simulink model "case3"  (R2024b)
settings: Solver=FixedStepAuto  StartTime=0  StopTime=1  FixedStep=1e-7  RelTol=1e-3
values from neighbouring files (symbols this model uses):
  SG_D_1_D = 0.01056    [IEEE9_case_parameters.m]    (also in case1_parameters.m; case2_parameters.m; case3_parameters.m; case4_parameters.m)
  SG_D_1_EnableSaturation = 0    [IEEE9_case_parameters.m]    (also in case1_parameters.m; case2_parameters.m; case3_parameters.m; case4_parameters.m)
  SG_D_1_f0 = 60    [IEEE9_case_parameters.m]    (also in case1_parameters.m; case2_parameters.m; case3_parameters.m; case4_parameters.m)
  SG_D_1_H = 7.5    [IEEE9_case_parameters.m]    (also in case1_parameters.m; case2_parameters.m; case3_parameters.m; case4_parameters.m)
  SG_D_1_K_A = 20    [IEEE9_case_parameters.m]    (also in case1_parameters.m; case2_parameters.m; case3_parameters.m; case4_parameters.m)
  SG_D_1_K_E = 1.000000e+1    (= 10)    [IEEE9_case_parameters.m]    (also in case1_parameters.m; case2_parameters.m; case3_parameters.m; case4_parameters.m)
  SG_D_1_K_F = 2.363    [IEEE9_case_parameters.m]    (also in case1_parameters.m; case2_parameters.m; case3_parameters.m; case4_parameters.m)
  SG_D_1_K_s = 0.5    [IEEE9_case_parameters.m]    (also in case1_parameters.m = 5; case2_parameters.m = 5; case3_parameters.m = 5; case4_parameters.m = 5)
  SG_D_1_R_a = 0.001088    [IEEE9_case_parameters.m]    (also in case1_parameters.m; case2_parameters.m; case3_parameters.m; case4_parameters.m)
  SG_D_1_S_A = 1    [IEEE9_case_parameters.m]    (also in case1_parameters.m; case2_parameters.m; case3_parameters.m; case4_parameters.m)
  SG_D_1_S_B = 0.103    [IEEE9_case_parameters.m]    (also in case1_parameters.m; case2_parameters.m; case3_parameters.m; case4_parameters.m)
  SG_D_1_S_N = 10.659857    [IEEE9_case_parameters.m]    (also in case1_parameters.m; case2_parameters.m; case3_parameters.m; case4_parameters.m)
  SG_D_1_SpeedPara = 200    [IEEE9_case_parameters.m]    (also in case1_parameters.m; case2_parameters.m; case3_parameters.m; case4_parameters.m)
  SG_D_1_T_0 = 0.720173    [IEEE9_case_parameters.m]    (also in case1_parameters.m = 0.755522; case2_parameters.m = 0.808931; case3_parameters.m = 0.869402; case4_parameters.m = 0.729316)
  SG_D_1_T_1 = 0.3    [IEEE9_case_parameters.m]    (also in case1_parameters.m; case2_parameters.m; case3_parameters.m; case4_parameters.m)
  SG_D_1_T_2 = 0.05    [IEEE9_case_parameters.m]    (also in case1_parameters.m; case2_parameters.m; case3_parameters.m; case4_parameters.m)
  SG_D_1_T_3 = 0.02    [IEEE9_case_parameters.m]    (also in case1_parameters.m; case2_parameters.m; case3_parameters.m; case4_parameters.m)
  SG_D_1_T_4 = 0.005    [IEEE9_case_parameters.m]    (also in case1_parameters.m; case2_parameters.m; case3_parameters.m; case4_parameters.m)
  SG_D_1_T_A = 0.02    [IEEE9_case_parameters.m]    (also in case1_parameters.m; case2_parameters.m; case3_parameters.m; case4_parameters.m)
  SG_D_1_T_dd = 8.000000e+0    (= 8)    [IEEE9_case_parameters.m]    (also in case1_parameters.m; case2_parameters.m; case3_parameters.m; case4_parameters.m)
  SG_D_1_T_ddd = 0.04    [IEEE9_case_parameters.m]    (also in case1_parameters.m; case2_parameters.m; case3_parameters.m; case4_parameters.m)
  SG_D_1_T_E = 0.314    [IEEE9_case_parameters.m]    (also in case1_parameters.m; case2_parameters.m; case3_parameters.m; case4_parameters.m)
  SG_D_1_T_F = 0.35    [IEEE9_case_parameters.m]    (also in case1_parameters.m; case2_parameters.m; case3_parameters.m; case4_parameters.m)
  SG_D_1_T_qd = 0.8    [IEEE9_case_parameters.m]    (also in case1_parameters.m; case2_parameters.m; case3_parameters.m; case4_parameters.m)
  SG_D_1_T_qdd = 0.02    [IEEE9_case_parameters.m]    (also in case1_parameters.m; case2_parameters.m; case3_parameters.m; case4_parameters.m)
  SG_D_1_T_speed = 0.1    [IEEE9_case_parameters.m]    (also in case1_parameters.m = 200; case2_parameters.m = 200; case3_parameters.m = 200; case4_parameters.m = 200)
  SG_D_1_T_w = 0.5    [IEEE9_case_parameters.m]    (also in case1_parameters.m; case2_parameters.m; case3_parameters.m; case4_parameters.m)
  SG_D_1_V_ref = 1.990276    [IEEE9_case_parameters.m]    (also in case1_parameters.m = 2.042296; case2_parameters.m = 2.051388; case3_parameters.m = 2.089584; case4_parameters.m = 2.01845)
  SG_D_1_w_ref = 376.991118    [IEEE9_case_parameters.m]    (also in case1_parameters.m; case2_parameters.m; case3_parameters.m; case4_parameters.m)
  SG_D_1_wb = 6.000000e+1    (= 60)    [IEEE9_case_parameters.m]    (also in case1_parameters.m; case2_parameters.m; case3_parameters.m; case4_parameters.m)
  SG_D_1_x_d = 1.9    [IEEE9_case_parameters.m]    (also in case1_parameters.m; case2_parameters.m; case3_parameters.m; case4_parameters.m)
  SG_D_1_x_dd = 0.302    [IEEE9_case_parameters.m]    (also in case1_parameters.m; case2_parameters.m; case3_parameters.m; case4_parameters.m)
  SG_D_1_x_ddd = 0.204    [IEEE9_case_parameters.m]    (also in case1_parameters.m; case2_parameters.m; case3_parameters.m; case4_parameters.m)
  SG_D_1_x_l = 0.05    [IEEE9_case_parameters.m]    (also in case1_parameters.m; case2_parameters.m; case3_parameters.m; case4_parameters.m)
  SG_D_1_x_q = 1.3    [IEEE9_case_parameters.m]    (also in case1_parameters.m; case2_parameters.m; case3_parameters.m; case4_parameters.m)
  SG_D_1_x_qd = 0.5    [IEEE9_case_parameters.m]    (also in case1_parameters.m; case2_parameters.m; case3_parameters.m; case4_parameters.m)
  SG_D_1_x_qdd = 0.3    [IEEE9_case_parameters.m]    (also in case1_parameters.m; case2_parameters.m; case3_parameters.m; case4_parameters.m)
  SG_D_2_D = 0.02    [IEEE9_case_parameters.m]    (also in case1_parameters.m; case2_parameters.m; case3_parameters.m; case4_parameters.m)
  SG_D_2_EnableSaturation = 0    [IEEE9_case_parameters.m]    (also in case1_parameters.m; case2_parameters.m; case3_parameters.m; case4_parameters.m)
  SG_D_2_f0 = 60    [IEEE9_case_parameters.m]    (also in case1_parameters.m; case2_parameters.m; case3_parameters.m; case4_parameters.m)
  SG_D_2_H = 8.000000e+0    (= 8)    [IEEE9_case_parameters.m]    (also in case1_parameters.m; case2_parameters.m; case3_parameters.m; case4_parameters.m)
  SG_D_2_K_A = 20    [IEEE9_case_parameters.m]    (also in case1_parameters.m; case2_parameters.m; case3_parameters.m; case4_parameters.m)
  SG_D_2_K_E = 1.000000e+1    (= 10)    [IEEE9_case_parameters.m]    (also in case1_parameters.m; case2_parameters.m; case3_parameters.m; case4_parameters.m)
  SG_D_2_K_F = 2.363    [IEEE9_case_parameters.m]    (also in case1_parameters.m; case2_parameters.m; case3_parameters.m; case4_parameters.m)
  SG_D_2_K_s = 0.5    [IEEE9_case_parameters.m]    (also in case1_parameters.m = 4; case2_parameters.m = 4; case3_parameters.m = 4; case4_parameters.m = 4)
  SG_D_2_R_a = 0.001088    [IEEE9_case_parameters.m]    (also in case1_parameters.m; case2_parameters.m; case3_parameters.m; case4_parameters.m)
  SG_D_2_S_A = 1    [IEEE9_case_parameters.m]    (also in case1_parameters.m; case2_parameters.m; case3_parameters.m; case4_parameters.m)
  SG_D_2_S_B = 0.103    [IEEE9_case_parameters.m]    (also in case1_parameters.m; case2_parameters.m; case3_parameters.m; case4_parameters.m)
  SG_D_2_S_N = 10.659857    [IEEE9_case_parameters.m]    (also in case1_parameters.m; case2_parameters.m; case3_parameters.m; case4_parameters.m)
  SG_D_2_SpeedPara = 200    [IEEE9_case_parameters.m]    (also in case1_parameters.m; case2_parameters.m; case3_parameters.m; case4_parameters.m)
  SG_D_2_T_0 = 1.632913    [IEEE9_case_parameters.m]    (also in case1_parameters.m = 1.632925; case2_parameters.m = 1.632915; case3_parameters.m = 1.632914; case4_parameters.m = 1.632927)
  SG_D_2_T_1 = 0.2    [IEEE9_case_parameters.m]    (also in case1_parameters.m; case2_parameters.m; case3_parameters.m; case4_parameters.m)
  SG_D_2_T_2 = 0.05    [IEEE9_case_parameters.m]    (also in case1_parameters.m; case2_parameters.m; case3_parameters.m; case4_parameters.m)
  SG_D_2_T_3 = 0.02    [IEEE9_case_parameters.m]    (also in case1_parameters.m; case2_parameters.m; case3_parameters.m; case4_parameters.m)
  SG_D_2_T_4 = 0.005    [IEEE9_case_parameters.m]    (also in case1_parameters.m; case2_parameters.m; case3_parameters.m; case4_parameters.m)
  SG_D_2_T_A = 0.02    [IEEE9_case_parameters.m]    (also in case1_parameters.m; case2_parameters.m; case3_parameters.m; case4_parameters.m)
  SG_D_2_T_dd = 7.9    [IEEE9_case_parameters.m]    (also in case1_parameters.m; case2_parameters.m; case3_parameters.m; case4_parameters.m)
  SG_D_2_T_ddd = 0.04    [IEEE9_case_parameters.m]    (also in case1_parameters.m; case2_parameters.m; case3_parameters.m; case4_parameters.m)
  SG_D_2_T_E = 0.314    [IEEE9_case_parameters.m]    (also in case1_parameters.m; case2_parameters.m; case3_parameters.m; case4_parameters.m)
  SG_D_2_T_F = 0.35    [IEEE9_case_parameters.m]    (also in case1_parameters.m; case2_parameters.m; case3_parameters.m; case4_parameters.m)
  SG_D_2_T_qd = 0.8    [IEEE9_case_parameters.m]    (also in case1_parameters.m; case2_parameters.m; case3_parameters.m; case4_parameters.m)
  SG_D_2_T_qdd = 0.015    [IEEE9_case_parameters.m]    (also in case1_parameters.m; case2_parameters.m; case3_parameters.m; case4_parameters.m)
  SG_D_2_T_speed = 0.1    [IEEE9_case_parameters.m]    (also in case1_parameters.m = 150; case2_parameters.m = 150; case3_parameters.m = 150; case4_parameters.m = 150)
  SG_D_2_T_w = 0.35    [IEEE9_case_parameters.m]    (also in case1_parameters.m; case2_parameters.m; case3_parameters.m; case4_parameters.m)
  SG_D_2_V_ref = 2.58547    [IEEE9_case_parameters.m]    (also in case1_parameters.m = 2.597896; case2_parameters.m = 2.587136; case3_parameters.m = 2.586042; case4_parameters.m = 2.599679)
  SG_D_2_w_ref = 376.991118    [IEEE9_case_parameters.m]    (also in case1_parameters.m; case2_parameters.m; case3_parameters.m; case4_parameters.m)
  SG_D_2_wb = 6.000000e+1    (= 60)    [IEEE9_case_parameters.m]    (also in case1_parameters.m; case2_parameters.m; case3_parameters.m; case4_parameters.m)
  SG_D_2_x_d = 1.8    [IEEE9_case_parameters.m]    (also in case1_parameters.m; case2_parameters.m; case3_parameters.m; case4_parameters.m)
  SG_D_2_x_dd = 0.302    [IEEE9_case_parameters.m]    (also in case1_parameters.m; case2_parameters.m; case3_parameters.m; case4_parameters.m)
  SG_D_2_x_ddd = 0.204    [IEEE9_case_parameters.m]    (also in case1_parameters.m; case2_parameters.m; case3_parameters.m; case4_parameters.m)
  SG_D_2_x_l = 0.05    [IEEE9_case_parameters.m]    (also in case1_parameters.m; case2_parameters.m; case3_parameters.m; case4_parameters.m)
  SG_D_2_x_q = 1.25    [IEEE9_case_parameters.m]    (also in case1_parameters.m; case2_parameters.m; case3_parameters.m; case4_parameters.m)
  SG_D_2_x_qd = 0.5    [IEEE9_case_parameters.m]    (also in case1_parameters.m; case2_parameters.m; case3_parameters.m; case4_parameters.m)
  SG_D_2_x_qdd = 0.3    [IEEE9_case_parameters.m]    (also in case1_parameters.m; case2_parameters.m; case3_parameters.m; case4_parameters.m)
  SG_D_3_D = 0.02    [IEEE9_case_parameters.m]    (also in case1_parameters.m; case2_parameters.m; case3_parameters.m; case4_parameters.m)
  SG_D_3_EnableSaturation = 0    [IEEE9_case_parameters.m]    (also in case1_parameters.m; case2_parameters.m; case3_parameters.m; case4_parameters.m)
  SG_D_3_f0 = 60    [IEEE9_case_parameters.m]    (also in case1_parameters.m; case2_parameters.m; case3_parameters.m; case4_parameters.m)
  SG_D_3_H = 7.7    [IEEE9_case_parameters.m]    (also in case1_parameters.m; case2_parameters.m; case3_parameters.m; case4_parameters.m)
  SG_D_3_K_A = 20    [IEEE9_case_parameters.m]    (also in case1_parameters.m; case2_parameters.m; case3_parameters.m; case4_parameters.m)
  SG_D_3_K_E = 1.000000e+1    (= 10)    [IEEE9_case_parameters.m]    (also in case1_parameters.m; case2_parameters.m; case3_parameters.m; case4_parameters.m)
  SG_D_3_K_F = 2.363    [IEEE9_case_parameters.m]    (also in case1_parameters.m; case2_parameters.m; case3_parameters.m; case4_parameters.m)
  SG_D_3_K_s = 0.2    [IEEE9_case_parameters.m]    (also in case1_parameters.m = 2; case2_parameters.m = 2; case3_parameters.m = 2; case4_parameters.m = 2)
  SG_D_3_R_a = 0.001088    [IEEE9_case_parameters.m]    (also in case1_parameters.m; case2_parameters.m; case3_parameters.m; case4_parameters.m)
  SG_D_3_S_A = 1    [IEEE9_case_parameters.m]    (also in case1_parameters.m; case2_parameters.m; case3_parameters.m; case4_parameters.m)
  SG_D_3_S_B = 0.103    [IEEE9_case_parameters.m]    (also in case1_parameters.m; case2_parameters.m; case3_parameters.m; case4_parameters.m)
  SG_D_3_S_N = 10.659857    [IEEE9_case_parameters.m]    (also in case1_parameters.m; case2_parameters.m; case3_parameters.m; case4_parameters.m)
  SG_D_3_SpeedPara = 200    [IEEE9_case_parameters.m]    (also in case1_parameters.m; case2_parameters.m; case3_parameters.m; case4_parameters.m)
  SG_D_3_T_0 = 0.850788    [IEEE9_case_parameters.m]    (also in case1_parameters.m = 0.850786; case2_parameters.m = 0.850787; case3_parameters.m; case4_parameters.m = 0.850786)
  SG_D_3_T_1 = 0.2    [IEEE9_case_parameters.m]    (also in case1_parameters.m; case2_parameters.m; case3_parameters.m; case4_parameters.m)
  SG_D_3_T_2 = 0.05    [IEEE9_case_parameters.m]    (also in case1_parameters.m; case2_parameters.m; case3_parameters.m; case4_parameters.m)
  SG_D_3_T_3 = 0.02    [IEEE9_case_parameters.m]    (also in case1_parameters.m; case2_parameters.m; case3_parameters.m; case4_parameters.m)
  SG_D_3_T_4 = 0.005    [IEEE9_case_parameters.m]    (also in case1_parameters.m; case2_parameters.m; case3_parameters.m; case4_parameters.m)
  SG_D_3_T_A = 0.02    [IEEE9_case_parameters.m]    (also in case1_parameters.m; case2_parameters.m; case3_parameters.m; case4_parameters.m)
  SG_D_3_T_dd = 8.1    [IEEE9_case_parameters.m]    (also in case1_parameters.m; case2_parameters.m; case3_parameters.m; case4_parameters.m)
  SG_D_3_T_ddd = 0.04    [IEEE9_case_parameters.m]    (also in case1_parameters.m; case2_parameters.m; case3_parameters.m; case4_parameters.m)
  SG_D_3_T_E = 0.314    [IEEE9_case_parameters.m]    (also in case1_parameters.m; case2_parameters.m; case3_parameters.m; case4_parameters.m)
  SG_D_3_T_F = 0.35    [IEEE9_case_parameters.m]    (also in case1_parameters.m; case2_parameters.m; case3_parameters.m; case4_parameters.m)
  SG_D_3_T_qd = 0.8    [IEEE9_case_parameters.m]    (also in case1_parameters.m; case2_parameters.m; case3_parameters.m; case4_parameters.m)
  SG_D_3_T_qdd = 0.015    [IEEE9_case_parameters.m]    (also in case1_parameters.m; case2_parameters.m; case3_parameters.m; case4_parameters.m)
  SG_D_3_T_speed = 0.1    [IEEE9_case_parameters.m]    (also in case1_parameters.m = 180; case2_parameters.m = 180; case3_parameters.m = 180; case4_parameters.m = 180)
  SG_D_3_T_w = 0.4    [IEEE9_case_parameters.m]    (also in case1_parameters.m; case2_parameters.m; case3_parameters.m; case4_parameters.m)
  SG_D_3_V_ref = 1.892727    [IEEE9_case_parameters.m]    (also in case1_parameters.m = 1.906439; case2_parameters.m = 1.895535; case3_parameters.m = 1.892105; case4_parameters.m = 1.906598)
  SG_D_3_w_ref = 376.991118    [IEEE9_case_parameters.m]    (also in case1_parameters.m; case2_parameters.m; case3_parameters.m; case4_parameters.m)
  SG_D_3_wb = 6.000000e+1    (= 60)    [IEEE9_case_parameters.m]    (also in case1_parameters.m; case2_parameters.m; case3_parameters.m; case4_parameters.m)
  SG_D_3_x_d = 1.85    [IEEE9_case_parameters.m]    (also in case1_parameters.m; case2_parameters.m; case3_parameters.m; case4_parameters.m)
  SG_D_3_x_dd = 0.302    [IEEE9_case_parameters.m]    (also in case1_parameters.m; case2_parameters.m; case3_parameters.m; case4_parameters.m)
  SG_D_3_x_ddd = 0.204    [IEEE9_case_parameters.m]    (also in case1_parameters.m; case2_parameters.m; case3_parameters.m; case4_parameters.m)
  SG_D_3_x_l = 0.05    [IEEE9_case_parameters.m]    (also in case1_parameters.m; case2_parameters.m; case3_parameters.m; case4_parameters.m)
  SG_D_3_x_q = 1.2    [IEEE9_case_parameters.m]    (also in case1_parameters.m; case2_parameters.m; case3_parameters.m; case4_parameters.m)
  SG_D_3_x_qd = 0.5    [IEEE9_case_parameters.m]    (also in case1_parameters.m; case2_parameters.m; case3_parameters.m; case4_parameters.m)
  SG_D_3_x_qdd = 0.3    [IEEE9_case_parameters.m]    (also in case1_parameters.m; case2_parameters.m; case3_parameters.m; case4_parameters.m)
(part 4 of 12)

== system case3/AC_1/d_vq_bus_7_block ==
  note: d_vq_bus_7 in case3
      | $2106.09563369148\,\mathrm{iq}_{\mathrm{bus},7}-376.991118430775\,\mathrm{vd}_{\mathrm{bus},7}$
      | Automatically generated on 2025-10-31 19:02:04 .
  Alge_iq_bus_7_9bcfd : Inport
  State_vd_bus_7_2341e : Inport  Port=2
  Constant_2106.09563369148_1523e : Constant  Value=2106.09563369148
  Constant_376.991118430775_cd95a : Constant  Value=376.991118430775
  Product_43391 : Product
  Product_ed048 : Product
  Subtract_00e21 : Sum  Inputs=+-
  Blockout_d_vq_bus_7_00412 : Outport
  wires:
  Constant_2106.09563369148_1523e/1 -> Product_ed048/1
  Product_43391/1 -> Subtract_00e21/2
  Alge_iq_bus_7_9bcfd/1 -> Product_ed048/2
  Constant_376.991118430775_cd95a/1 -> Product_43391/1
  Subtract_00e21/1 -> Blockout_d_vq_bus_7_00412/1
  State_vd_bus_7_2341e/1 -> Product_43391/2
  Product_ed048/1 -> Subtract_00e21/1

== system case3/AC_1/d_vq_bus_8_block ==
  note: d_vq_bus_8 in case3
      | $1657.10381727813\,\mathrm{iq}_{\mathrm{bus},8}-376.991118430775\,\mathrm{vd}_{\mathrm{bus},8}$
      | Automatically generated on 2025-10-31 19:02:06 .
  Alge_iq_bus_8_0043b : Inport
  State_vd_bus_8_4778f : Inport  Port=2
  Constant_1657.10381727813_76750 : Constant  Value=1657.10381727813
  Constant_376.991118430775_a4e06 : Constant  Value=376.991118430775
  Product_09aa2 : Product
  Product_80b30 : Product
  Subtract_72ad1 : Sum  Inputs=+-
  Blockout_d_vq_bus_8_7125c : Outport
  wires:
  Constant_1657.10381727813_76750/1 -> Product_09aa2/1
  Constant_376.991118430775_a4e06/1 -> Product_80b30/1
  Alge_iq_bus_8_0043b/1 -> Product_09aa2/2
  State_vd_bus_8_4778f/1 -> Product_80b30/2
  Product_09aa2/1 -> Subtract_72ad1/1
  Product_80b30/1 -> Subtract_72ad1/2
  Subtract_72ad1/1 -> Blockout_d_vq_bus_8_7125c/1

== system case3/AC_1/d_vq_bus_9_block ==
  note: d_vq_bus_9 in case3
      | $1564.27849971276\,\mathrm{iq}_{\mathrm{bus},9}-376.991118430775\,\mathrm{vd}_{\mathrm{bus},9}$
      | Automatically generated on 2025-10-31 19:02:07 .
  Alge_iq_bus_9_e4ae9 : Inport
  State_vd_bus_9_0824c : Inport  Port=2
  Constant_1564.27849971276_a5fe3 : Constant  Value=1564.27849971276
  Constant_376.991118430775_65cab : Constant  Value=376.991118430775
  Product_26de2 : Product
  Product_50707 : Product
  Subtract_bc7f1 : Sum  Inputs=+-
  Blockout_d_vq_bus_9_e5b12 : Outport
  wires:
  Constant_1564.27849971276_a5fe3/1 -> Product_50707/1
  Constant_376.991118430775_65cab/1 -> Product_26de2/1
  Alge_iq_bus_9_e4ae9/1 -> Product_50707/2
  State_vd_bus_9_0824c/1 -> Product_26de2/2
  Product_50707/1 -> Subtract_bc7f1/1
  Product_26de2/1 -> Subtract_bc7f1/2
  Subtract_bc7f1/1 -> Blockout_d_vq_bus_9_e5b12/1

== system case3/AC_1/id_bus_1_block ==
  note: id_bus_1 in case3
      | $\mathrm{id}_{\mathrm{SG},D,1}-\mathrm{id}_{\mathrm{line},1,4}$
      | Automatically generated on 2025-10-31 19:02:38 .
  Input_id_SG_D_1_696b1 : Inport
  State_id_line_1_4_e72f3 : Inport  Port=2
  Subtract_53e99 : Sum  Inputs=+-
  Blockout_id_bus_1_4a65c : Outport
  wires:
  Input_id_SG_D_1_696b1/1 -> Subtract_53e99/1
  State_id_line_1_4_e72f3/1 -> Subtract_53e99/2
  Subtract_53e99/1 -> Blockout_id_bus_1_4a65c/1

== system case3/AC_1/id_bus_2_block ==
  note: id_bus_2 in case3
      | $\mathrm{id}_{\mathrm{SG},D,2}+\mathrm{id}_{\mathrm{line},8,2}$
      | Automatically generated on 2025-10-31 19:02:40 .
  Input_id_SG_D_2_bafef : Inport
  State_id_line_8_2_6b5a6 : Inport  Port=2
  Add_c2829 : Sum
  Blockout_id_bus_2_bddd5 : Outport
  wires:
  Input_id_SG_D_2_bafef/1 -> Add_c2829/1
  State_id_line_8_2_6b5a6/1 -> Add_c2829/2
  Add_c2829/1 -> Blockout_id_bus_2_bddd5/1

== system case3/AC_1/id_bus_3_block ==
  note: id_bus_3 in case3
      | $\mathrm{id}_{\mathrm{SG},D,3}-\mathrm{id}_{\mathrm{line},3,6}$
      | Automatically generated on 2025-10-31 19:02:43 .
  Input_id_SG_D_3_6c44f : Inport
  State_id_line_3_6_571a6 : Inport  Port=2
  Subtract_f2fe0 : Sum  Inputs=+-
  Blockout_id_bus_3_5b536 : Outport
  wires:
  Input_id_SG_D_3_6c44f/1 -> Subtract_f2fe0/1
  State_id_line_3_6_571a6/1 -> Subtract_f2fe0/2
  Subtract_f2fe0/1 -> Blockout_id_bus_3_5b536/1

== system case3/AC_1/id_bus_4_block ==
  note: id_bus_4 in case3
      | $\mathrm{id}_{\mathrm{line},1,4}-\mathrm{id}_{\mathrm{line},4,5}+\mathrm{id}_{\mathrm{line},9,4}$
      | Automatically generated on 2025-10-31 19:02:44 .
  State_id_line_1_4_bd9f3 : Inport
  State_id_line_4_5_71002 : Inport  Port=2
  State_id_line_9_4_dd8eb : Inport  Port=3
  Add_de6d1 : Sum
  Subtract_ec270 : Sum  Inputs=+-
  Blockout_id_bus_4_47d2f : Outport
  wires:
  State_id_line_9_4_dd8eb/1 -> Add_de6d1/2
  State_id_line_1_4_bd9f3/1 -> Subtract_ec270/1
  State_id_line_4_5_71002/1 -> Subtract_ec270/2
  Subtract_ec270/1 -> Add_de6d1/1
  Add_de6d1/1 -> Blockout_id_bus_4_47d2f/1

== system case3/AC_1/id_bus_5_block ==
  note: id_bus_5 in case3
      | $\mathrm{id}_{\mathrm{line},4,5}-\mathrm{id}_{\mathrm{load},5}-\mathrm{id}_{\mathrm{line},5,6}$
      | Automatically generated on 2025-10-31 19:02:46 .
  State_id_load_5_b6667 : Inport
  State_id_line_4_5_78e66 : Inport  Port=2
  State_id_line_5_6_8fb3f : Inport  Port=3
  Add_36a5e : Sum
  Constant_-1_8506f : Constant  Value=-1
  Product_690f2 : Product
  Subtract_ac2bb : Sum  Inputs=+-
  Blockout_id_bus_5_0f46c : Outport
  wires:
  Subtract_ac2bb/1 -> Blockout_id_bus_5_0f46c/1
  State_id_line_4_5_78e66/1 -> Add_36a5e/2
  Constant_-1_8506f/1 -> Product_690f2/1
  Add_36a5e/1 -> Subtract_ac2bb/1
  State_id_load_5_b6667/1 -> Product_690f2/2
  Product_690f2/1 -> Add_36a5e/1
  State_id_line_5_6_8fb3f/1 -> Subtract_ac2bb/2

== system case3/AC_1/id_bus_6_block ==
  note: id_bus_6 in case3
      | $\mathrm{id}_{\mathrm{line},3,6}+\mathrm{id}_{\mathrm{line},5,6}-\mathrm{id}_{\mathrm{line},6,7}$
      | Automatically generated on 2025-10-31 19:02:47 .
  State_id_line_3_6_c6af3 : Inport
  State_id_line_5_6_cc1e8 : Inport  Port=2
  State_id_line_6_7_32134 : Inport  Port=3
  Add_59c7e : Sum
  Subtract_31bf1 : Sum  Inputs=+-
  Blockout_id_bus_6_05d15 : Outport
  wires:
  State_id_line_6_7_32134/1 -> Subtract_31bf1/2
  State_id_line_3_6_c6af3/1 -> Add_59c7e/1
  State_id_line_5_6_cc1e8/1 -> Add_59c7e/2
  Add_59c7e/1 -> Subtract_31bf1/1
  Subtract_31bf1/1 -> Blockout_id_bus_6_05d15/1

== system case3/AC_1/id_bus_7_block ==
  note: id_bus_7 in case3
      | $\mathrm{id}_{\mathrm{line},6,7}-\mathrm{id}_{\mathrm{load},7}-\mathrm{id}_{\mathrm{line},7,8}$
      | Automatically generated on 2025-10-31 19:02:49 .
  State_id_load_7_37f76 : Inport
  State_id_line_6_7_64680 : Inport  Port=2
  State_id_line_7_8_85cde : Inport  Port=3
  Add_ba5f6 : Sum
  Constant_-1_f6e4f : Constant  Value=-1
  Product_2a424 : Product
  Subtract_4cf74 : Sum  Inputs=+-
  Blockout_id_bus_7_20b6b : Outport
  wires:
  Subtract_4cf74/1 -> Blockout_id_bus_7_20b6b/1
  State_id_line_6_7_64680/1 -> Add_ba5f6/2
  Constant_-1_f6e4f/1 -> Product_2a424/1
  Add_ba5f6/1 -> Subtract_4cf74/1
  State_id_load_7_37f76/1 -> Product_2a424/2
  Product_2a424/1 -> Add_ba5f6/1
  State_id_line_7_8_85cde/1 -> Subtract_4cf74/2

== system case3/AC_1/id_bus_8_block ==
  note: id_bus_8 in case3
      | $\mathrm{id}_{\mathrm{line},7,8}-\mathrm{id}_{\mathrm{line},8,2}-\mathrm{id}_{\mathrm{line},8,9}$
      | Automatically generated on 2025-10-31 19:02:51 .
  State_id_line_7_8_e2cc9 : Inport
  State_id_line_8_2_3e7ba : Inport  Port=2
  State_id_line_8_9_302ee : Inport  Port=3
  Subtract_27381 : Sum  Inputs=+-
  Subtract_b9667 : Sum  Inputs=+-
  Blockout_id_bus_8_01350 : Outport
  wires:
  State_id_line_8_9_302ee/1 -> Subtract_b9667/2
  State_id_line_7_8_e2cc9/1 -> Subtract_27381/1
  State_id_line_8_2_3e7ba/1 -> Subtract_27381/2
  Subtract_27381/1 -> Subtract_b9667/1
  Subtract_b9667/1 -> Blockout_id_bus_8_01350/1

== system case3/AC_1/id_bus_9_block ==
  note: id_bus_9 in case3
      | $\mathrm{id}_{\mathrm{line},8,9}-\mathrm{id}_{\mathrm{load},9}-\mathrm{id}_{\mathrm{line},9,4}$
      | Automatically generated on 2025-10-31 19:02:52 .
  State_id_load_9_08adc : Inport
  State_id_line_8_9_ceed5 : Inport  Port=2
  State_id_line_9_4_1728f : Inport  Port=3
  Add_64fa5 : Sum
  Constant_-1_2f2f1 : Constant  Value=-1
  Product_af254 : Product
  Subtract_1fc9b : Sum  Inputs=+-
  Blockout_id_bus_9_70dbc : Outport
  wires:
  Subtract_1fc9b/1 -> Blockout_id_bus_9_70dbc/1
  State_id_line_8_9_ceed5/1 -> Add_64fa5/2
  Constant_-1_2f2f1/1 -> Product_af254/1
  Add_64fa5/1 -> Subtract_1fc9b/1
  State_id_load_9_08adc/1 -> Product_af254/2
  Product_af254/1 -> Add_64fa5/1
  State_id_line_9_4_1728f/1 -> Subtract_1fc9b/2

== system case3/AC_1/iq_bus_1_block ==
  note: iq_bus_1 in case3
      | $\mathrm{iq}_{\mathrm{SG},D,1}-\mathrm{iq}_{\mathrm{line},1,4}$
      | Automatically generated on 2025-10-31 19:02:38 .
  Input_iq_SG_D_1_691df : Inport
  State_iq_line_1_4_8b10a : Inport  Port=2
  Subtract_bf583 : Sum  Inputs=+-
  Blockout_iq_bus_1_cefb8 : Outport
  wires:
  Input_iq_SG_D_1_691df/1 -> Subtract_bf583/1
  State_iq_line_1_4_8b10a/1 -> Subtract_bf583/2
  Subtract_bf583/1 -> Blockout_iq_bus_1_cefb8/1

== system case3/AC_1/iq_bus_2_block ==
  note: iq_bus_2 in case3
      | $\mathrm{iq}_{\mathrm{SG},D,2}+\mathrm{iq}_{\mathrm{line},8,2}$
      | Automatically generated on 2025-10-31 19:02:41 .
  Input_iq_SG_D_2_ed99c : Inport
  State_iq_line_8_2_3621d : Inport  Port=2
  Add_92b39 : Sum
  Blockout_iq_bus_2_c2560 : Outport
  wires:
  Input_iq_SG_D_2_ed99c/1 -> Add_92b39/1
  State_iq_line_8_2_3621d/1 -> Add_92b39/2
  Add_92b39/1 -> Blockout_iq_bus_2_c2560/1

== system case3/AC_1/iq_bus_3_block ==
  note: iq_bus_3 in case3
      | $\mathrm{iq}_{\mathrm{SG},D,3}-\mathrm{iq}_{\mathrm{line},3,6}$
      | Automatically generated on 2025-10-31 19:02:43 .
  Input_iq_SG_D_3_dee65 : Inport
  State_iq_line_3_6_61dd2 : Inport  Port=2
  Subtract_e728d : Sum  Inputs=+-
  Blockout_iq_bus_3_7f48b : Outport
  wires:
  Input_iq_SG_D_3_dee65/1 -> Subtract_e728d/1
  State_iq_line_3_6_61dd2/1 -> Subtract_e728d/2
  Subtract_e728d/1 -> Blockout_iq_bus_3_7f48b/1

== system case3/AC_1/iq_bus_4_block ==
  note: iq_bus_4 in case3
      | $\mathrm{iq}_{\mathrm{line},1,4}-\mathrm{iq}_{\mathrm{line},4,5}+\mathrm{iq}_{\mathrm{line},9,4}$
      | Automatically generated on 2025-10-31 19:02:45 .
  State_iq_line_1_4_b88bb : Inport
  State_iq_line_4_5_adb37 : Inport  Port=2
  State_iq_line_9_4_3e12c : Inport  Port=3
  Add_1fb56 : Sum
  Subtract_2b2df : Sum  Inputs=+-
  Blockout_iq_bus_4_14ae7 : Outport
  wires:
  State_iq_line_1_4_b88bb/1 -> Subtract_2b2df/1
  State_iq_line_4_5_adb37/1 -> Subtract_2b2df/2
  Subtract_2b2df/1 -> Add_1fb56/1
  State_iq_line_9_4_3e12c/1 -> Add_1fb56/2
  Add_1fb56/1 -> Blockout_iq_bus_4_14ae7/1

== system case3/AC_1/iq_bus_5_block ==
  note: iq_bus_5 in case3
      | $\mathrm{iq}_{\mathrm{line},4,5}-\mathrm{iq}_{\mathrm{load},5}-\mathrm{iq}_{\mathrm{line},5,6}$
      | Automatically generated on 2025-10-31 19:02:47 .
  State_iq_load_5_2754d : Inport
  State_iq_line_4_5_89bcd : Inport  Port=2
  State_iq_line_5_6_c4019 : Inport  Port=3
  Add_c4d41 : Sum
  Constant_-1_2f333 : Constant  Value=-1
  Product_39ca3 : Product
  Subtract_68927 : Sum  Inputs=+-
  Blockout_iq_bus_5_d6d28 : Outport
  wires:
  Subtract_68927/1 -> Blockout_iq_bus_5_d6d28/1
  State_iq_line_4_5_89bcd/1 -> Add_c4d41/2
  Constant_-1_2f333/1 -> Product_39ca3/1
  State_iq_load_5_2754d/1 -> Product_39ca3/2
  Product_39ca3/1 -> Add_c4d41/1
  Add_c4d41/1 -> Subtract_68927/1
  State_iq_line_5_6_c4019/1 -> Subtract_68927/2

== system case3/AC_1/iq_bus_6_block ==
  note: iq_bus_6 in case3
      | $\mathrm{iq}_{\mathrm{line},3,6}+\mathrm{iq}_{\mathrm{line},5,6}-\mathrm{iq}_{\mathrm{line},6,7}$
      | Automatically generated on 2025-10-31 19:02:48 .
  State_iq_line_3_6_33d27 : Inport
  State_iq_line_5_6_019c6 : Inport  Port=2
  State_iq_line_6_7_054b0 : Inport  Port=3
  Add_d3aef : Sum
  Subtract_4e3ec : Sum  Inputs=+-
  Blockout_iq_bus_6_95ebc : Outport
  wires:
  State_iq_line_3_6_33d27/1 -> Add_d3aef/1
  State_iq_line_5_6_019c6/1 -> Add_d3aef/2
  Add_d3aef/1 -> Subtract_4e3ec/1
  State_iq_line_6_7_054b0/1 -> Subtract_4e3ec/2
  Subtract_4e3ec/1 -> Blockout_iq_bus_6_95ebc/1

== system case3/AC_1/iq_bus_7_block ==
  note: iq_bus_7 in case3
      | $\mathrm{iq}_{\mathrm{line},6,7}-\mathrm{iq}_{\mathrm{load},7}-\mathrm{iq}_{\mathrm{line},7,8}$
      | Automatically generated on 2025-10-31 19:02:50 .
  State_iq_load_7_960e8 : Inport
  State_iq_line_6_7_03f81 : Inport  Port=2
  State_iq_line_7_8_95be5 : Inport  Port=3
  Add_47c7b : Sum
  Constant_-1_469e3 : Constant  Value=-1
  Product_518e4 : Product
  Subtract_c0759 : Sum  Inputs=+-
  Blockout_iq_bus_7_bb486 : Outport
  wires:
  Subtract_c0759/1 -> Blockout_iq_bus_7_bb486/1
  State_iq_line_6_7_03f81/1 -> Add_47c7b/2
  Constant_-1_469e3/1 -> Product_518e4/1
  State_iq_load_7_960e8/1 -> Product_518e4/2
  Product_518e4/1 -> Add_47c7b/1
  Add_47c7b/1 -> Subtract_c0759/1
  State_iq_line_7_8_95be5/1 -> Subtract_c0759/2

== system case3/AC_1/iq_bus_8_block ==
  note: iq_bus_8 in case3
      | $\mathrm{iq}_{\mathrm{line},7,8}-\mathrm{iq}_{\mathrm{line},8,2}-\mathrm{iq}_{\mathrm{line},8,9}$
      | Automatically generated on 2025-10-31 19:02:51 .
  State_iq_line_7_8_0aaeb : Inport
  State_iq_line_8_2_60ac3 : Inport  Port=2
  State_iq_line_8_9_6619f : Inport  Port=3
  Subtract_54fe6 : Sum  Inputs=+-
  Subtract_93871 : Sum  Inputs=+-
  Blockout_iq_bus_8_33408 : Outport
  wires:
  State_iq_line_7_8_0aaeb/1 -> Subtract_54fe6/1
  State_iq_line_8_2_60ac3/1 -> Subtract_54fe6/2
  Subtract_54fe6/1 -> Subtract_93871/1
  State_iq_line_8_9_6619f/1 -> Subtract_93871/2
  Subtract_93871/1 -> Blockout_iq_bus_8_33408/1

== system case3/AC_1/iq_bus_9_block ==
  note: iq_bus_9 in case3
      | $\mathrm{iq}_{\mathrm{line},8,9}-\mathrm{iq}_{\mathrm{load},9}-\mathrm{iq}_{\mathrm{line},9,4}$
      | Automatically generated on 2025-10-31 19:02:53 .
  State_iq_load_9_56201 : Inport
  State_iq_line_8_9_f042c : Inport  Port=2
  State_iq_line_9_4_00fae : Inport  Port=3
  Add_29842 : Sum
  Constant_-1_51dab : Constant  Value=-1
  Product_ccf99 : Product
  Subtract_5ae72 : Sum  Inputs=+-
  Blockout_iq_bus_9_4e4a2 : Outport
  wires:
  Subtract_5ae72/1 -> Blockout_iq_bus_9_4e4a2/1
  State_iq_line_8_9_f042c/1 -> Add_29842/2
  Constant_-1_51dab/1 -> Product_ccf99/1
  State_iq_load_9_56201/1 -> Product_ccf99/2
  Product_ccf99/1 -> Add_29842/1
  Add_29842/1 -> Subtract_5ae72/1
  State_iq_line_9_4_00fae/1 -> Subtract_5ae72/2

== system case3/AC_1/vd_bus_1_out_block ==
  note: vd_bus_1_out in case3
      | $\mathrm{vd}_{\mathrm{bus},1}$
      | Automatically generated on 2025-10-31 19:02:37 .
  State_vd_bus_1_379f4 : Inport
  Blockout_vd_bus_1_out_2faa7 : Outport
  wires:
  State_vd_bus_1_379f4/1 -> Blockout_vd_bus_1_out_2faa7/1

== system case3/AC_1/vd_bus_2_out_block ==
  note: vd_bus_2_out in case3
      | $\mathrm{vd}_{\mathrm{bus},2}$
      | Automatically generated on 2025-10-31 19:02:39 .
  State_vd_bus_2_2714d : Inport
  Blockout_vd_bus_2_out_79f6a : Outport
  wires:
  State_vd_bus_2_2714d/1 -> Blockout_vd_bus_2_out_79f6a/1

== system case3/AC_1/vd_bus_3_out_block ==
  note: vd_bus_3_out in case3
      | $\mathrm{vd}_{\mathrm{bus},3}$
      | Automatically generated on 2025-10-31 19:02:41 .
  State_vd_bus_3_9218c : Inport
  Blockout_vd_bus_3_out_036f2 : Outport
  wires:
  State_vd_bus_3_9218c/1 -> Blockout_vd_bus_3_out_036f2/1

== system case3/AC_1/vq_bus_1_out_block ==
  note: vq_bus_1_out in case3
      | $\mathrm{vq}_{\mathrm{bus},1}$
      | Automatically generated on 2025-10-31 19:02:37 .
  State_vq_bus_1_ac5cf : Inport
  Blockout_vq_bus_1_out_b4fc0 : Outport
  wires:
  State_vq_bus_1_ac5cf/1 -> Blockout_vq_bus_1_out_b4fc0/1

== system case3/AC_1/vq_bus_2_out_block ==
  note: vq_bus_2_out in case3
      | $\mathrm{vq}_{\mathrm{bus},2}$
      | Automatically generated on 2025-10-31 19:02:39 .
  State_vq_bus_2_9d425 : Inport
  Blockout_vq_bus_2_out_740a9 : Outport
  wires:
  State_vq_bus_2_9d425/1 -> Blockout_vq_bus_2_out_740a9/1

== system case3/AC_1/vq_bus_3_out_block ==
  note: vq_bus_3_out in case3
      | $\mathrm{vq}_{\mathrm{bus},3}$
      | Automatically generated on 2025-10-31 19:02:42 .
  State_vq_bus_3_4ba96 : Inport
  Blockout_vq_bus_3_out_fa0c1 : Outport
  wires:
  State_vq_bus_3_4ba96/1 -> Blockout_vq_bus_3_out_fa0c1/1

== system case3/SG_D_1/T_e_SG_D_1_block ==
  note: T_e_SG_D_1 in case3
      | $-\frac{\psi _{d,\mathrm{SG},D,1}\,\left(\psi _{q,\mathrm{SG},D,1}+\frac{\psi _{\mathrm{gq},\mathrm{SG},D,1}\,\left(x_{l}-x_{\mathrm{qdd}}\right)}{x_{l}-x_{\mathrm{qd}}}+\frac{\psi _{\mathrm{kq},\mathrm{SG},D,1}\,\left(x_{\mathrm{qd}}-x_{\mathrm{qdd}}\right)}{x_{l}-x_{\mathrm{qd}}}\right)}{x_{\mathrm{qdd}}}-\frac{\psi _{q,\mathrm{SG},D,1}\,\left(\frac{\psi _{\mathrm{1d},\mathrm{SG},D,1}\,\left(x_{\mathrm{dd}}-x_{\mathrm{ddd}}\right)}{x_{\mathrm{dd}}-x_{l}}-\psi _{d,\mathrm{SG},D,1}+\frac{\psi _{\mathrm{fd},\mathrm{SG},D,1}\,\left(x_{\mathrm{ddd}}-x_{l}\right)}{x_{\mathrm{dd}}-x_{l}}\right)}{x_{\mathrm{ddd}}}$
      | Automatically generated on 2025-10-31 18:59:38 .
  State_psi_d_SG_D_1_3a885 : Inport
  State_psi_gq_SG_D_1_4e0b7 : Inport  Port=2
  State_psi_kq_SG_D_1_043c6 : Inport  Port=3
  State_psi_q_SG_D_1_aebda : Inport  Port=4
  State_psi_q_SG_D_1_dfa5e : Inport  Port=5
  State_psi_1d_SG_D_1_26ac5 : Inport  Port=6
  State_psi_d_SG_D_1_bdeee : Inport  Port=7
  State_psi_fd_SG_D_1_be33b : Inport  Port=8
  Add_4ec82 : Sum
  Add_5b24a : Sum
  Add_91b02 : Sum
  Add_c6c73 : Sum
  Add_e3b63 : Sum
  Add_f678f : Sum
  Constant_-1_01abd : Constant  Value=-1
  Constant_-1_35de7 : Constant  Value=-1
  Constant_-1_5cc00 : Constant  Value=-1
  Constant_-1_65d39 : Constant  Value=-1
  Constant_-1_84c0a : Constant  Value=-1
  Constant_x_dd_18510 : Constant  Value=x_dd
  Constant_x_dd_5496d : Constant  Value=x_dd
  Constant_x_dd_d85de : Constant  Value=x_dd
  Constant_x_ddd_47183 : Constant  Value=x_ddd
  Constant_x_ddd_c8fe4 : Constant  Value=x_ddd
  Constant_x_ddd_f910b : Constant  Value=x_ddd
  Constant_x_l_31d57 : Constant  Value=x_l
  Constant_x_l_6d9aa : Constant  Value=x_l
  Constant_x_l_8a284 : Constant  Value=x_l
  Constant_x_l_9e89d : Constant  Value=x_l
  Constant_x_l_d36b2 : Constant  Value=x_l
  Constant_x_l_fceac : Constant  Value=x_l
  Constant_x_qd_5c7e4 : Constant  Value=x_qd
  Constant_x_qd_9d2e4 : Constant  Value=x_qd
  Constant_x_qd_c5a39 : Constant  Value=x_qd
  Constant_x_qdd_3382f : Constant  Value=x_qdd
  Constant_x_qdd_caa63 : Constant  Value=x_qdd
  Constant_x_qdd_da2d9 : Constant  Value=x_qdd
  Divide_1106d : Product  Inputs=*/
  Divide_668bf : Product  Inputs=*/
  Divide_829ec : Product  Inputs=*/
  Divide_aa027 : Product  Inputs=*/
  Divide_b9ff5 : Product  Inputs=*/
  Divide_bad9d : Product  Inputs=*/
  Product_033c2 : Product
  Product_158d6 : Product
  Product_22fde : Product
  Product_37ac9 : Product
  Product_6c65f : Product
  Product_9515b : Product
  Product_9d9b8 : Product
  Product_ae37e : Product
  Product_f1624 : Product
  Product_f51cc : Product
  Product_f9cf8 : Product
  Subtract_08213 : Sum  Inputs=+-
  Subtract_591c7 : Sum  Inputs=+-
  Subtract_6c762 : Sum  Inputs=+-
  Subtract_b4e4f : Sum  Inputs=+-
  Subtract_d466a : Sum  Inputs=+-
  Subtract_f046a : Sum  Inputs=+-
  Subtract_fcb1b : Sum  Inputs=+-
  Blockout_T_e_SG_D_1_96ef2 : Outport
  wires:
  Product_37ac9/1 -> Divide_b9ff5/1
  Product_033c2/1 -> Add_e3b63/1
  Divide_b9ff5/1 -> Subtract_fcb1b/1
  Constant_-1_35de7/1 -> Product_033c2/1
  Constant_x_l_d36b2/1 -> Product_033c2/2
  Constant_x_qdd_3382f/1 -> Add_e3b63/2
  Constant_x_qd_c5a39/1 -> Subtract_b4e4f/1
  Constant_-1_01abd/1 -> Product_158d6/1
  Constant_x_qdd_caa63/1 -> Divide_829ec/2
  Constant_x_qdd_da2d9/1 -> Subtract_b4e4f/2
  State_psi_q_SG_D_1_dfa5e/1 -> Product_f1624/1
  Constant_x_dd_d85de/1 -> Subtract_591c7/1
  Constant_x_l_6d9aa/1 -> Product_158d6/2
  Subtract_591c7/1 -> Product_9d9b8/2
  Constant_-1_5cc00/1 -> Product_22fde/1
  Constant_x_l_fceac/1 -> Product_22fde/2
  Subtract_d466a/1 -> Product_f1624/2
  State_psi_q_SG_D_1_aebda/1 -> Add_f678f/2
  Constant_-1_84c0a/1 -> Product_6c65f/1
  State_psi_1d_SG_D_1_26ac5/1 -> Product_6c65f/2
  Constant_x_ddd_f910b/1 -> Subtract_591c7/2
  State_psi_gq_SG_D_1_4e0b7/1 -> Product_37ac9/1
  Add_e3b63/1 -> Product_37ac9/2
  Product_158d6/1 -> Add_5b24a/1
  Product_f51cc/1 -> Product_9515b/1
  Constant_x_qd_5c7e4/1 -> Add_5b24a/2
  Product_9d9b8/1 -> Divide_1106d/1
  State_psi_kq_SG_D_1_043c6/1 -> Product_ae37e/1
  Add_5b24a/1 -> Divide_b9ff5/2
  Subtract_b4e4f/1 -> Product_ae37e/2
  Product_22fde/1 -> Add_91b02/1
  Constant_x_qd_9d2e4/1 -> Add_91b02/2
  Product_ae37e/1 -> Divide_bad9d/1
  Product_6c65f/1 -> Product_9d9b8/1
  Constant_x_dd_5496d/1 -> Subtract_6c762/1
  Constant_x_l_8a284/1 -> Subtract_6c762/2
  Constant_x_ddd_47183/1 -> Subtract_08213/1
  Product_f1624/1 -> Divide_aa027/1
  Constant_x_l_31d57/1 -> Subtract_08213/2
  Divide_829ec/1 -> Add_c6c73/1
  Product_9515b/1 -> Divide_829ec/1
  Add_91b02/1 -> Divide_bad9d/2
  Subtract_fcb1b/1 -> Add_f678f/1
  Divide_bad9d/1 -> Subtract_fcb1b/2
  Subtract_6c762/1 -> Divide_1106d/2
  State_psi_fd_SG_D_1_be33b/1 -> Product_f9cf8/1
  Constant_x_ddd_c8fe4/1 -> Divide_aa027/2
  Subtract_08213/1 -> Product_f9cf8/2
  Constant_x_dd_18510/1 -> Subtract_f046a/1
  Constant_x_l_9e89d/1 -> Subtract_f046a/2
  Divide_1106d/1 -> Add_4ec82/1
  Add_4ec82/1 -> Subtract_d466a/1
  State_psi_d_SG_D_1_bdeee/1 -> Add_4ec82/2
  Product_f9cf8/1 -> Divide_668bf/1
  Subtract_f046a/1 -> Divide_668bf/2
  Constant_-1_65d39/1 -> Product_f51cc/1
  State_psi_d_SG_D_1_3a885/1 -> Product_f51cc/2
  Divide_668bf/1 -> Subtract_d466a/2
  Add_f678f/1 -> Product_9515b/2
  Divide_aa027/1 -> Add_c6c73/2
  Add_c6c73/1 -> Blockout_T_e_SG_D_1_96ef2/1

== system case3/SG_D_1/d_E_fd_SG_D_1_block ==
  note: d_E_fd_SG_D_1 in case3
      | $\frac{V_{f,\mathrm{SG},D,1}-E_{\mathrm{fd},\mathrm{SG},D,1}\,K_{E}}{T_{E}}$
      | Automatically generated on 2025-10-31 18:59:21 .
  State_E_fd_SG_D_1_54b5a : Inport
  State_V_f_SG_D_1_a5ff7 : Inport  Port=2
  Add_08a00 : Sum
  Constant_-1_7bc5b : Constant  Value=-1
  Constant_K_E_4ad97 : Constant  Value=K_E
  Constant_T_E_0652c : Constant  Value=T_E
  Divide_c4753 : Product  Inputs=*/
  Product_67673 : Product
  Product_b682e : Product
  Blockout_d_E_fd_SG_D_1_6015a : Outport
  wires:
  Add_08a00/1 -> Divide_c4753/1
  Constant_-1_7bc5b/1 -> Product_67673/1
  State_E_fd_SG_D_1_54b5a/1 -> Product_67673/2
  Product_67673/1 -> Product_b682e/1
  Constant_K_E_4ad97/1 -> Product_b682e/2
  Product_b682e/1 -> Add_08a00/1
  Constant_T_E_0652c/1 -> Divide_c4753/2
  State_V_f_SG_D_1_a5ff7/1 -> Add_08a00/2
  Divide_c4753/1 -> Blockout_d_E_fd_SG_D_1_6015a/1

== system case3/SG_D_1/d_Px_1_SG_D_1_block ==
  note: d_Px_1_SG_D_1 in case3
      | $\frac{w_{\mathrm{SG},D,1}-2\,\pi \,f_{0}}{T_{w}}-\frac{\mathrm{Px}_{1,\mathrm{SG},D,1}}{T_{w}}$
      | Automatically generated on 2025-10-31 18:59:22 .
  State_Px_1_SG_D_1_be173 : Inport
  State_w_SG_D_1_918fc : Inport  Port=2
  Add_6ff8d : Sum
  Add_8e171 : Sum
  Constant_-1_5656d : Constant  Value=-1
  Constant_-2.0_2a3a5 : Constant  Value=-2.0
  Constant_T_w_19ac2 : Constant  Value=T_w
  Constant_T_w_ccb4a : Constant  Value=T_w
  Constant_f0_c6ec4 : Constant  Value=f0
  Constant_pi_b6a6d : Constant  Value=pi
  Divide_6e725 : Product  Inputs=*/
  Divide_805cf : Product  Inputs=*/
  Product_59a6d : Product
  Product_a0621 : Product
  Product_a6fc9 : Product
  Blockout_d_Px_1_SG_D_1_2cd45 : Outport
  wires:
  Add_8e171/1 -> Blockout_d_Px_1_SG_D_1_2cd45/1
  Constant_-2.0_2a3a5/1 -> Product_59a6d/1
  Product_a6fc9/1 -> Divide_6e725/1
  State_w_SG_D_1_918fc/1 -> Add_6ff8d/2
  Constant_-1_5656d/1 -> Product_a6fc9/1
  Constant_f0_c6ec4/1 -> Product_a0621/2
  Constant_pi_b6a6d/1 -> Product_59a6d/2
  Product_a0621/1 -> Add_6ff8d/1
  Product_59a6d/1 -> Product_a0621/1
  State_Px_1_SG_D_1_be173/1 -> Product_a6fc9/2
  Constant_T_w_19ac2/1 -> Divide_6e725/2
  Add_6ff8d/1 -> Divide_805cf/1
  Constant_T_w_ccb4a/1 -> Divide_805cf/2
  Divide_6e725/1 -> Add_8e171/1
  Divide_805cf/1 -> Add_8e171/2

== system case3/SG_D_1/d_Px_2_SG_D_1_block ==
  note: d_Px_2_SG_D_1 in case3
      | $\frac{\mathrm{Px}_{1,\mathrm{SG},D,1}-T_{2}\,\left(\frac{\mathrm{Px}_{1,\mathrm{SG},D,1}}{T_{w}}-\frac{w_{\mathrm{SG},D,1}-2\,\pi \,f_{0}}{T_{w}}\right)}{T_{1}}-\frac{\mathrm{Px}_{2,\mathrm{SG},D,1}}{T_{1}}$
      | Automatically generated on 2025-10-31 18:59:24 .
  State_Px_2_SG_D_1_f7c33 : Inport
  State_Px_1_SG_D_1_0d618 : Inport  Port=2
  State_Px_1_SG_D_1_e9c5b : Inport  Port=3
  State_w_SG_D_1_5fb1d : Inport  Port=4
  Add_13b84 : Sum
  Add_3eea4 : Sum
  Add_a7158 : Sum
  Add_b9494 : Sum
  Constant_-1_c63ee : Constant  Value=-1
  Constant_-1_dce67 : Constant  Value=-1
  Constant_-2.0_7bb93 : Constant  Value=-2.0
  Constant_T_1_09492 : Constant  Value=T_1
  Constant_T_1_ff0e5 : Constant  Value=T_1
  Constant_T_2_cf1f1 : Constant  Value=T_2
  Constant_T_w_7e51f : Constant  Value=T_w
  Constant_T_w_f051d : Constant  Value=T_w
  Constant_f0_bfcfc : Constant  Value=f0
  Constant_pi_7b062 : Constant  Value=pi
  Divide_2ef5d : Product  Inputs=*/
  Divide_d917d : Product  Inputs=*/
  Divide_dca93 : Product  Inputs=*/
  Divide_e897c : Product  Inputs=*/
  Product_4d230 : Product
  Product_b0528 : Product
  Product_cc9e9 : Product
  Product_e60b2 : Product
  Product_f98e8 : Product
  Blockout_d_Px_2_SG_D_1_b732b : Outport
  wires:
  Constant_-2.0_7bb93/1 -> Product_b0528/1
  State_w_SG_D_1_5fb1d/1 -> Add_b9494/2
  Constant_f0_bfcfc/1 -> Product_e60b2/2
  Constant_pi_7b062/1 -> Product_b0528/2
  Add_a7158/1 -> Product_cc9e9/2
  Product_e60b2/1 -> Add_b9494/1
  Divide_e897c/1 -> Add_a7158/1
  Product_b0528/1 -> Product_e60b2/1
  Constant_T_w_7e51f/1 -> Divide_e897c/2
  Constant_-1_dce67/1 -> Product_f98e8/1
  State_Px_1_SG_D_1_e9c5b/1 -> Product_f98e8/2
  Divide_2ef5d/1 -> Add_13b84/1
  Product_f98e8/1 -> Divide_e897c/1
  Add_b9494/1 -> Divide_d917d/1
  Constant_T_w_f051d/1 -> Divide_d917d/2
  Divide_d917d/1 -> Add_a7158/2
  Constant_T_2_cf1f1/1 -> Product_cc9e9/1
  Constant_-1_c63ee/1 -> Product_4d230/1
  State_Px_2_SG_D_1_f7c33/1 -> Product_4d230/2
  State_Px_1_SG_D_1_0d618/1 -> Add_3eea4/1
  Product_cc9e9/1 -> Add_3eea4/2
  Add_3eea4/1 -> Divide_dca93/1
  Product_4d230/1 -> Divide_2ef5d/1
  Constant_T_1_09492/1 -> Divide_2ef5d/2
  Constant_T_1_ff0e5/1 -> Divide_dca93/2
  Divide_dca93/1 -> Add_13b84/2
  Add_13b84/1 -> Blockout_d_Px_2_SG_D_1_b732b/1

== system case3/SG_D_1/d_Px_3_SG_D_1_block ==
  note: d_Px_3_SG_D_1 in case3
      | $\frac{\mathrm{Px}_{2,\mathrm{SG},D,1}+T_{4}\,\left(\frac{\mathrm{Px}_{1,\mathrm{SG},D,1}-T_{2}\,\left(\frac{\mathrm{Px}_{1,\mathrm{SG},D,1}}{T_{w}}-\frac{w_{\mathrm{SG},D,1}-2\,\pi \,f_{0}}{T_{w}}\right)}{T_{1}}-\frac{\mathrm{Px}_{2,\mathrm{SG},D,1}}{T_{1}}\right)}{T_{3}}-\frac{\mathrm{Px}_{3,\mathrm{SG},D,1}}{T_{3}}$
      | Automatically generated on 2025-10-31 18:59:26 .
  State_Px_3_SG_D_1_48de8 : Inport
  State_Px_2_SG_D_1_d9c58 : Inport  Port=2
  State_Px_2_SG_D_1_c3f1d : Inport  Port=3
  State_Px_1_SG_D_1_0dee8 : Inport  Port=4
  State_Px_1_SG_D_1_09b4d : Inport  Port=5
  State_w_SG_D_1_8f01a : Inport  Port=6
  Add_01fb5 : Sum
  Add_199d2 : Sum
  Add_455a8 : Sum
  Add_4be50 : Sum
  Add_6b97f : Sum
  Add_dc92d : Sum
  Constant_-1_6840d : Constant  Value=-1
  Constant_-1_c8e7b : Constant  Value=-1
  Constant_-1_d4ce2 : Constant  Value=-1
  Constant_-2.0_e03fb : Constant  Value=-2.0
  Constant_T_1_4eb1d : Constant  Value=T_1
  Constant_T_1_6eeca : Constant  Value=T_1
  Constant_T_2_5722d : Constant  Value=T_2
  Constant_T_3_bb900 : Constant  Value=T_3
  Constant_T_3_f7683 : Constant  Value=T_3
  Constant_T_4_5897d : Constant  Value=T_4
  Constant_T_w_36749 : Constant  Value=T_w
  Constant_T_w_fe27f : Constant  Value=T_w
  Constant_f0_8a46f : Constant  Value=f0
  Constant_pi_6e96c : Constant  Value=pi
  Divide_20fdf : Product  Inputs=*/
  Divide_32743 : Product  Inputs=*/
  Divide_3d31f : Product  Inputs=*/
  Divide_9e2c3 : Product  Inputs=*/
  Divide_c510c : Product  Inputs=*/
  Divide_d347e : Product  Inputs=*/
  Product_396e2 : Product
  Product_72677 : Product
  Product_980c5 : Product
  Product_b2ff5 : Product
  Product_e26bd : Product
  Product_e3e9b : Product
  Product_eed95 : Product
  Blockout_d_Px_3_SG_D_1_c155d : Outport
  wires:
  Constant_T_w_fe27f/1 -> Divide_32743/2
  Constant_-1_c8e7b/1 -> Product_b2ff5/1
  Add_6b97f/1 -> Blockout_d_Px_3_SG_D_1_c155d/1
  Constant_-2.0_e03fb/1 -> Product_980c5/1
  State_w_SG_D_1_8f01a/1 -> Add_4be50/2
  Constant_f0_8a46f/1 -> Product_e26bd/2
  State_Px_1_SG_D_1_09b4d/1 -> Product_b2ff5/2
  Constant_pi_6e96c/1 -> Product_980c5/2
  Product_e26bd/1 -> Add_4be50/1
  Product_980c5/1 -> Product_e26bd/1
  Product_b2ff5/1 -> Divide_32743/1
  Divide_9e2c3/1 -> Add_6b97f/1
  Constant_T_3_bb900/1 -> Divide_d347e/2
  Add_4be50/1 -> Divide_3d31f/1
  Constant_T_w_36749/1 -> Divide_3d31f/2
  Divide_32743/1 -> Add_dc92d/1
  Divide_3d31f/1 -> Add_dc92d/2
  Constant_-1_6840d/1 -> Product_72677/1
  Constant_T_2_5722d/1 -> Product_e3e9b/1
  Add_dc92d/1 -> Product_e3e9b/2
  Constant_-1_d4ce2/1 -> Product_eed95/1
  Divide_d347e/1 -> Add_6b97f/2
  Constant_T_3_f7683/1 -> Divide_9e2c3/2
  State_Px_2_SG_D_1_c3f1d/1 -> Product_eed95/2
  State_Px_1_SG_D_1_0dee8/1 -> Add_01fb5/1
  Divide_c510c/1 -> Add_455a8/1
  Product_e3e9b/1 -> Add_01fb5/2
  Product_eed95/1 -> Divide_c510c/1
  Product_72677/1 -> Divide_9e2c3/1
  Constant_T_1_6eeca/1 -> Divide_c510c/2
  Add_01fb5/1 -> Divide_20fdf/1
  Constant_T_1_4eb1d/1 -> Divide_20fdf/2
  Divide_20fdf/1 -> Add_455a8/2
  Constant_T_4_5897d/1 -> Product_396e2/1
  Add_455a8/1 -> Product_396e2/2
  State_Px_3_SG_D_1_48de8/1 -> Product_72677/2
  State_Px_2_SG_D_1_d9c58/1 -> Add_199d2/1
  Product_396e2/1 -> Add_199d2/2
  Add_199d2/1 -> Divide_d347e/1

== system case3/SG_D_1/d_R_f_SG_D_1_block ==
  note: d_R_f_SG_D_1 in case3
      | $-\frac{R_{f,\mathrm{SG},D,1}-\frac{E_{\mathrm{fd},\mathrm{SG},D,1}\,K_{F}}{T_{F}}}{T_{F}}$
      | Automatically generated on 2025-10-31 18:59:20 .
  State_E_fd_SG_D_1_a064f : Inport
  State_R_f_SG_D_1_95d12 : Inport  Port=2
  Constant_K_F_c43e2 : Constant  Value=K_F
  Constant_T_F_ea69e : Constant  Value=T_F
  Constant_T_F_f579f : Constant  Value=T_F
  Divide_08728 : Product  Inputs=*/
  Divide_89d95 : Product  Inputs=*/
  Product_024be : Product
  Subtract_d7bd2 : Sum  Inputs=+-
  Blockout_d_R_f_SG_D_1_eadac : Outport
  wires:
  Constant_K_F_c43e2/1 -> Product_024be/2
  Product_024be/1 -> Divide_08728/1
  State_E_fd_SG_D_1_a064f/1 -> Product_024be/1
  State_R_f_SG_D_1_95d12/1 -> Subtract_d7bd2/2
  Constant_T_F_f579f/1 -> Divide_08728/2
  Divide_08728/1 -> Subtract_d7bd2/1
  Divide_89d95/1 -> Blockout_d_R_f_SG_D_1_eadac/1
  Subtract_d7bd2/1 -> Divide_89d95/1
  Constant_T_F_ea69e/1 -> Divide_89d95/2

== system case3/SG_D_1/d_T_m_SG_D_1_block ==
  note: d_T_m_SG_D_1 in case3
      | $-\frac{T_{m,\mathrm{SG},D,1}-T_{0}+\frac{\mathrm{SpeedPara}\,\left(w_{\mathrm{SG},D,1}-w_{\mathrm{ref}}\right)}{2\,f_{0}\,\pi }}{T_{\mathrm{speed}}}$
      | Automatically generated on 2025-10-31 18:59:11 .
  State_w_SG_D_1_82698 : Inport
  State_T_m_SG_D_1_b9754 : Inport  Port=2
  Add_acde0 : Sum
  Add_fd255 : Sum
  Constant_-1_49282 : Constant  Value=-1
  Constant_2.0_f9a59 : Constant  Value=2.0
  Constant_SpeedPara_01d26 : Constant  Value=SpeedPara
  Constant_T_0_352e8 : Constant  Value=T_0
  Constant_T_speed_ccca7 : Constant  Value=T_speed
  Constant_f0_c178b : Constant  Value=f0
  Constant_pi_b1d7e : Constant  Value=pi
  Constant_w_ref_773e4 : Constant  Value=w_ref
  Divide_d54f1 : Product  Inputs=*/
  Divide_e4a8b : Product  Inputs=*/
  Product_53581 : Product
  Product_61f54 : Product
  Product_a1660 : Product
  Product_a4025 : Product
  Subtract_4861c : Sum  Inputs=+-
  Blockout_d_T_m_SG_D_1_21740 : Outport
  wires:
  Constant_-1_49282/1 -> Product_53581/1
  Constant_w_ref_773e4/1 -> Add_fd255/2
  State_w_SG_D_1_82698/1 -> Product_53581/2
  Add_acde0/1 -> Subtract_4861c/1
  Add_fd255/1 -> Product_a4025/2
  Product_53581/1 -> Add_fd255/1
  Constant_2.0_f9a59/1 -> Product_a1660/1
  Constant_pi_b1d7e/1 -> Product_a1660/2
  Constant_SpeedPara_01d26/1 -> Product_a4025/1
  Product_a1660/1 -> Product_61f54/1
  Constant_f0_c178b/1 -> Product_61f54/2
  Constant_T_speed_ccca7/1 -> Divide_d54f1/2
  Product_a4025/1 -> Divide_e4a8b/1
  Product_61f54/1 -> Divide_e4a8b/2
  Divide_e4a8b/1 -> Add_acde0/1
  Constant_T_0_352e8/1 -> Add_acde0/2
  State_T_m_SG_D_1_b9754/1 -> Subtract_4861c/2
  Subtract_4861c/1 -> Divide_d54f1/1
  Divide_d54f1/1 -> Blockout_d_T_m_SG_D_1_21740/1
